simulink model "power_3phPWM3level"  (Simulink 6.0)
settings: Solver=FixedStepDiscrete  SolverMode=SingleTasking  StartTime=0.0  StopTime=0.1  FixedStep=Ts  RelTol=1e-3
InitFcn:
  | assignin('base','Ts',[1/60/3240])
undefined symbols (not defined in the file or in its folder): level, Ts
libraries: powerlib x13, powerlib_extras x3
settings Model: Creator=hyp01  LastModifiedBy=batserve  ExtModeTrigMode=oneshot  ExtModeArmWhenConnect=off  ExtModeAutoUpdateStatusClock=off
settings DataIOCC: LimitDataPoints=off  SaveOutput=off  SaveTime=off  SignalLoggingName=sigsOut
settings OptimizationCC: BlockReduction=off  BooleanDataType=off
settings DebuggingCC: CheckExecutionContextPreStartOutputMsg=on  CheckExecutionContextRuntimeOutputMsg=on  SolverPrmCheckMsg=none
settings HardwareCC: TargetUnknown=on

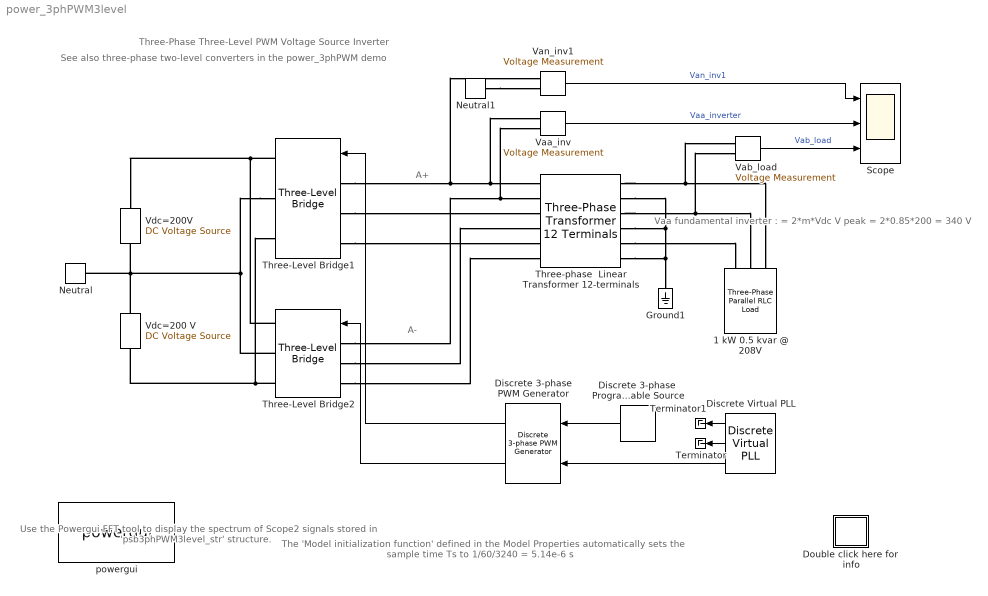
== system power_3phPWM3level ==
  note: Vaa fundamental inverter :
      | = 2*m*Vdc V peak
      | = 2*0.85*200
      | = 340 V
  note: Three-Phase Three-Level PWM Voltage Source Inverter
  note: See also three-phase two-level converters in the power_3phPWM demo
  note: Use the Powergui FFT tool to display
      | the spectrum of Scope2  signals stored
      | in 'psb3phPWM3level_str' structure.
  note: A+
  note: A-
  note: The 'Model  initialization function' defined in the
      | Model Properties automatically sets the sample time Ts
      | to 1/60/3240 = 5.14e-6 s
  "  Vdc=200 V" : powerlib/Electrical Sources/DC Voltage Source  Description=source block  Orientation=up  Amplitude=200  Measurements=None
      settings: AttributesFormatString=\n
  "1 kW 0.5 kvar @ 208V " : powerlib/Elements/Three-Phase Parallel RLC Load  Orientation=down  PhysicalDomain=powersysdomain  SubClassName=unknown  LeftPortType=p1  RightPortType=p1  LConnTagsString=A|B|C  Configuration=Y (grounded)  NominalVoltage=208  NominalFrequency=60  ActivePower=1000  InductivePower=0  CapacitivePower=500  Measurements=None
  Discrete 3-phase  Programmable Source : powerlib_extras/Discrete  Control Blocks/Discrete 3-phase  Programmable Source  Orientation=left  Par_Vps=[0.85 0 60]  VariationEntity=None  VariationType=Step  VariationStep=-0.5  VariationRate=10  VariationMag=0.3  VariationFreq=2  Par_Timing_Variation=[0.1 1.2]  SinglePhase=on  Yampli=[1 0.2 1.2 1.0]  Xtime=[0 0.1 0.15 0.2]  HarmonicGeneration=off  Par_HarmoA=[3 0.2 -25 0]  Par_HarmoB=[2 0.15 35 2]  Par_Timing_Harmo="[0.05  3]"  Ts=Ts
  Discrete Virtual PLL : powerlib_extras/Discrete  Control Blocks/Discrete Virtual PLL  Orientation=left  Freq=60  Phase=0  Ts=Ts
  Discrete 3-phase PWM Generator : powerlib_extras/Discrete  Control Blocks/Discrete 3-phase PWM Generator  Orientation=left  ModulatorType=3-level  ModulatorMode=Synchronized  nF=18  Fc=18*60  ModulatingSignals=off  m=0.85  Freq=60  Phase=0  Ts=Ts
  Double click here for  info : Subsystem
      mask Display: disp('?')
  Ground1 : powerlib/Elements/Ground  Orientation=down  PhysicalDomain=powersysdomain  SubClassName=unknown  LeftPortType=p1  RightPortType=p1  LConnTagsString=a
  Neutral : powerlib/Elements/Neutral  Orientation=left  PhysicalDomain=powersysdomain  SubClassName=unknown  LeftPortType=p1  RightPortType=p1  LConnTagsString=a  RConnTagsString=__newr0  NodeNumber=10
  Neutral1 : powerlib/Elements/Neutral  Orientation=left  PhysicalDomain=powersysdomain  SubClassName=unknown  LeftPortType=p1  RightPortType=p1  LConnTagsString=a  RConnTagsString=__newr0  NodeNumber=10
  Scope : Scope  NumInputPorts=3
      settings: TimeRange=0.1  YMin=-300~-400~-400  YMax=300~400~400  SaveName=psb3phPWM3level_str  MaxDataPoints=500000
  Terminator : Terminator
  Terminator1 : Terminator
  Three-Level Bridge1 : powerlib/Power Electronics/Three-Level Bridge  Orientation=left  Arms=3  SnubberResistance=1e6  SbubberCapacitance=inf  Device=GTO / Diodes  Ron=1e-4  ForwardVoltages="[  1  1  ]"  Measurements=None
  Three-Level Bridge2 : powerlib/Power Electronics/Three-Level Bridge  Orientation=left  Arms=3  SnubberResistance=1e6  SbubberCapacitance=inf  Device=GTO / Diodes  Ron=1e-4  ForwardVoltages="[  1  1  ]"  Measurements=None
  Three-phase  Linear Transformer 12-terminals : powerlib/Elements/Three-Phase Transformer 12 Terminals  RatedPower=[ 1000 60 ]  Winding1="[ 240  0.002  0.04 ]"  Winding2=[ 208/sqrt(3) 0.002 0.04]  RmXm=[ 200 200 ]
      settings: AttributesFormatString=\n
  Vaa_inv : powerlib/Measurements/Voltage Measurement  Tag=PoWeRsYsTeMmEaSuReMeNt  PhasorSimulation=off  OutputType=Magnitude  PSBequivalent=0
  Vab_load : powerlib/Measurements/Voltage Measurement  Tag=PoWeRsYsTeMmEaSuReMeNt  PhasorSimulation=off  OutputType=Magnitude  PSBequivalent=0
  Van_inv1 : powerlib/Measurements/Voltage Measurement  Tag=PoWeRsYsTeMmEaSuReMeNt  PhasorSimulation=off  OutputType=Magnitude  PSBequivalent=0
  "Vdc=200V " : powerlib/Electrical Sources/DC Voltage Source  Description=source block  Orientation=up  Amplitude=200  Measurements=None
      settings: AttributesFormatString=\n
  powergui : powerlib/powergui  Priority=2  Frange=[0:2:500]  Ylog=off  Xlog=off  save=off  variable=ZData  structure=psb3phPWM3level_str  ZoomFFT=on  StartTime=0.1-2/60  cycles=2  DisplayStyle=off  fundamental=60  FreqAxis=on  MaxFrequency=5000  frequencyindice=1  frequencyindicesteady=1  RmsSteady=1  display=off  Ts=Ts  methode=off  frequency=60  echomessages=on
  wires:
  Discrete Virtual PLL/1 -> Terminator1/1
  Discrete Virtual PLL/2 -> Terminator/1
  Discrete 3-phase  Programmable Source/1 -> Discrete 3-phase PWM Generator/1
  Discrete Virtual PLL/3 -> Discrete 3-phase PWM Generator/2
  Vab_load/1 -> Scope/3  "Vab_load"
  Van_inv1/1 -> Scope/1  "Van_inv1"
  Vaa_inv/1 -> Scope/2  "Vaa_inverter"
  Discrete 3-phase PWM Generator/1 -> Three-Level Bridge1/1
  Discrete 3-phase PWM Generator/2 -> Three-Level Bridge2/1
  connections:
  Three-phase  Linear Transformer 12-terminals/RConn1 -- Vab_load/LConn1 -- "1 kW 0.5 kvar @ 208V "/LConn3
  Three-Level Bridge1/LConn1 -- Van_inv1/LConn1 -- Vaa_inv/LConn1 -- Three-phase  Linear Transformer 12-terminals/LConn1
  Three-Level Bridge1/LConn2 -- Three-phase  Linear Transformer 12-terminals/LConn3
  Three-Level Bridge1/LConn3 -- Three-phase  Linear Transformer 12-terminals/LConn5
  Three-Level Bridge2/LConn1 -- Vaa_inv/LConn2 -- Three-phase  Linear Transformer 12-terminals/LConn2
  Three-Level Bridge2/LConn2 -- Three-phase  Linear Transformer 12-terminals/LConn4
  Three-Level Bridge2/LConn3 -- Three-phase  Linear Transformer 12-terminals/LConn6
  Three-phase  Linear Transformer 12-terminals/RConn3 -- Vab_load/LConn2 -- "1 kW 0.5 kvar @ 208V "/LConn2
  Three-phase  Linear Transformer 12-terminals/RConn5 -- "1 kW 0.5 kvar @ 208V "/LConn1
  Three-phase  Linear Transformer 12-terminals/RConn4 -- Three-phase  Linear Transformer 12-terminals/RConn2 -- Ground1/LConn1 -- Three-phase  Linear Transformer 12-terminals/RConn6
  Three-Level Bridge1/RConn1 -- "Vdc=200V "/RConn1 -- Three-Level Bridge2/RConn1
  Three-Level Bridge2/RConn3 -- Three-Level Bridge1/RConn3 -- "  Vdc=200 V"/LConn1
  Three-Level Bridge1/RConn2 -- Three-Level Bridge2/RConn2 -- "  Vdc=200 V"/RConn1 -- "Vdc=200V "/LConn1 -- Neutral/LConn1
  Neutral1/LConn1 -- Van_inv1/LConn2

== system power_3phPWM3level/Double click here for  info ==
  note: This demonstration illustrates simulation of a 3-phase, 3-level inverter
      | and Discrete 3-phase PWM Generator. It also demonstrates
      | harmonic analysis of PWM waveforms using the Powergui/FFT tool.
  note: Circuit Description
  note: Demonstration
  note: P. Giroux and G. Sybille (Hydro-Quebec)
  note: Run the simulation and observe the following three waveforms on the Scope block:
      | Phase-neutral voltage Van_inv1 generated by  inverter 1 (trace 1), phase A voltage Vaa_inverter generated by the twin inverter (trace 2) and
      | phase-phase load voltage Vab_load (trace 3). The Van_inv1 waveform cleary demonstrates the three levels:  +200 V, 0 V, and -200 V.
      |
      | Once the  simulation is completed, open the Powergui and select  'FFT Analysis' to display the 0 - 5000 Hz frequency spectrum of signals saved
      | in the 'psb3phPWM3level_str' structure. The FFT will be performed on  a 2-cycle window starting at t = 0.1 - 2/60 (last 2 cycles of recording).
      | Selelect the input labeled 'Vaa _inverter'. Click on Display and observe the frequency spectrum of last 2 cycles.
      |
      | The fundamental component of  Vaa_inverter and THD for the 0 - 5000 Hz frequency range are displayed above the spectrum window.
      | Because of the forward voltage drops in the IGBTs (Vf=1 V) and diodes (Vfd=1V), the magnitude of the fundamental voltage of the inverter (335 V)
      | is slightly lower than the theoretical value (340 V for m=0.85). As expected for a twin inverter, first harmonics occur around multiples of double
      | of carrier frequency (n*2*1080 Hz +- k*60Hz).
      |
      | The same circuit using  two-level inverters in twin configuration is available in the psb3phPWM.mdl demonstration file.
      | Run this demo and compare the harmonic contents in the 2-level and 3-level inverter  voltage for the same modulation index (m = 0.85).
      | Harmonics occur at the same frequencies but their magnitude is approximately two times lower for a 3-level inverter.
  note: The system consists of two three-phase three-level PWM voltage source converters connected in twin configuration
      | The  inverter feeds an AC load (1kW, 500 var 60Hz @ 208 Vrms) through a three-phase transformer.
      | Harmonic filtering is performed by the transformer leakage inductance (8%) and load capacitance (500 var).
      |
      | Each of the two inverters uses the Three-Level Bridge block where the specified power electronic devices are IGBT/Diode pairs.
      | Each arm consists of 4 IGBTs, 4 antiparallel diodes, and 2 neutral clamping diodes.
      |
      | The inverter is controlled in open loop. Pulses are generated by the Discrete 3-Phase Discrete PWM Generator block. This block is available in the
      | Extras/Discrete Control Blocks library. This PWM generator or modulator can be used to generate pulses for 3-phase, 2-level, or 3-level converters using
      | one bridge or two bridges (twin configuration). In this demo, the PWM modulator generates two sets of 12 pulses (1 set per inverter) at P1 and P2 outputs.
      | Open the 'Discrete 3-phase PWM Generator' menu. Notice that the generator can operate either in synchronized or un-synchronized mode.
      | When operating in synchronized mode, the carrier triangular signal is synchronized on a PLL reference angle connected to input 'wt'.
      | In synchronized mode, the carrier chopping frequency is specified by the switching ratio as a multiple of the output frequency.
      |
      | Three sinusoidal 0.85 pu modulating signals are provided by the 'Discrete 3-phase Programmable Source' to obtain a modulation index  of 0.85.
      | The carrier signals are synchronized on the modulating signals. in the PWM Generator block, you can instead select  'Un-synchronized' and
      | 'Internal generation of modulating signals'. In such a case the magnitude (modulation index), frequency and phase angle of the output signals
      | are specified. directly inside the PWM Generator block menu.
      |
      | For this example the DC bus voltage is  400V (+/- 200 V) , chopping  frequency is 1080 Hz (18*60 Hz), magnitude of  the three modulating signals is 0.85
      | (corresponding to a modulation index  m = 0.85) and the frequency of the three generated signals is 60 Hz.
      |
      | In order to allow further signal processing, signals displayed on the Scope block  (sampled at simulation sampling rate of 3240 samples/ cycle)
      | are stored in a variable named 'psb3phPWM3level_str'  (structures with time) .
